simulink model "LAB"  (R2023a)
settings: Solver=VariableStepAuto  StartTime=0.0  StopTime=10.0  RelTol=1e-3
undefined symbols (not defined in the file): T
settings Model: Creator=Mohamed Ezzelrgal  LastModifiedBy=Mohamed Ezzelrgal

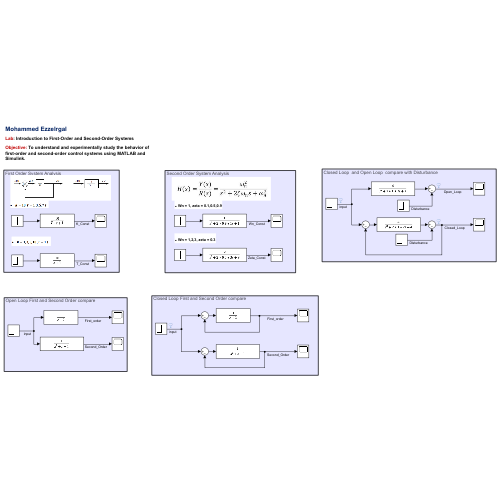
[thumbnail: Simulink's stored preview of the top-level diagram]
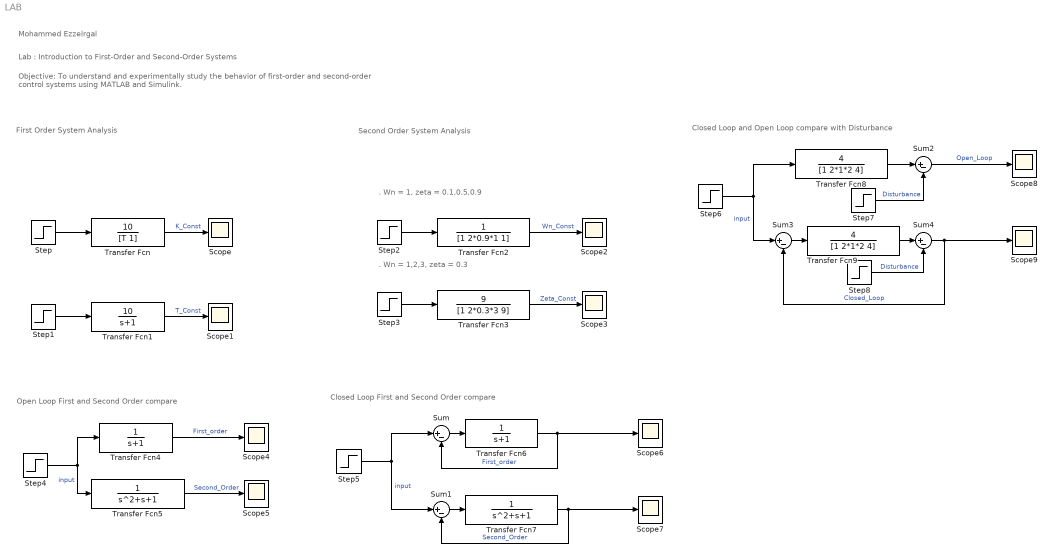
== system LAB ==
  note: Closed Loop First and Second Order compare
  note: Open Loop First and Second Order compare
  note: Second Order System Analysis
  note: . Wn = 1, zeta = 0.1,0.5,0.9
  note: First Order System Analysis
  note: Mohammed Ezzelrgal
  note: Objective: To understand and experimentally study the behavior of first-order and second-order control systems using MATLAB and Simulink.
  note: Lab : Introduction to First-Order and Second-Order Systems
  note: . Wn = 1,2,3, zeta = 0.3
  note: Closed Loop and Open Loop compare with Disturbance
  Scope{,1..9} (10 alike) : Scope
  Step{,1..6} (7 alike) : Step  SampleTime=0
  Step7 : Step  Time=3  After=1.2  SampleTime=0
  Step8 : Step  Time=3  After=1.2  SampleTime=0
  Sum{,1..4} (5 alike) : Sum  Inputs=|+-
  Transfer Fcn : TransferFcn  Numerator=[10]  Denominator=[T 1]
  Transfer Fcn1 : TransferFcn  Numerator=[10]  Denominator=[1 1]
  Transfer Fcn2 : TransferFcn  Denominator=[1 2*0.9*1 1]
  Transfer Fcn3 : TransferFcn  Numerator=[9]  Denominator=[1 2*0.3*3 9]
  Transfer Fcn4 : TransferFcn  Denominator=[1 1]
  Transfer Fcn5 : TransferFcn  Denominator=[1 1 1]
  Transfer Fcn6 : TransferFcn  Denominator=[1 1]
  Transfer Fcn7 : TransferFcn  Denominator=[1 1 1]
  Transfer Fcn8 : TransferFcn  Numerator=[4]  Denominator=[1 2*1*2 4]
  Transfer Fcn9 : TransferFcn  Numerator=[4]  Denominator=[1 2*1*2 4]
  wires:
  Step/1 -> Transfer Fcn/1
  Transfer Fcn/1 -> Scope/1  "K_Const"
  Transfer Fcn1/1 -> Scope1/1  "T_Const"
  Step1/1 -> Transfer Fcn1/1
  Transfer Fcn2/1 -> Scope2/1  "Wn_Const"
  Step2/1 -> Transfer Fcn2/1
  Step3/1 -> Transfer Fcn3/1
  Transfer Fcn3/1 -> Scope3/1  "Zeta_Const"
  Transfer Fcn4/1 -> Scope4/1  "First_order"
  Step4/1 -> Transfer Fcn4/1, Transfer Fcn5/1  "input"
  Transfer Fcn5/1 -> Scope5/1  "Second_Order"
  Transfer Fcn7/1 -> Sum1/2, Scope7/1  "Second_Order"
  Transfer Fcn6/1 -> Scope6/1, Sum/2  "First_order"
  Sum/1 -> Transfer Fcn6/1
  Step5/1 -> Sum1/1, Sum/1  "input"
  Sum1/1 -> Transfer Fcn7/1
  Sum3/1 -> Transfer Fcn9/1
  Step6/1 -> Transfer Fcn8/1, Sum3/1  "input"
  Transfer Fcn8/1 -> Sum2/1
  Sum2/1 -> Scope8/1  "Open_Loop"
  Step7/1 -> Sum2/2  "Disturbance"
  Transfer Fcn9/1 -> Sum4/1
  Sum4/1 -> Scope9/1, Sum3/2  "Closed_Loop"
  Step8/1 -> Sum4/2  "Disturbance"
